simulink model "Polynominal"  (R2019b)
settings: Solver=ode1  StartTime=0.0  StopTime=Inf  FixedStep=0.001  RelTol=1e-3
PostLoadFcn:
  | , if any(exist('dsrtsu_mdlpostloadfcn', 'file') == [2, 3, 6]), try dsrtsu_mdlpostloadfcn('Execute', bdroot); catch fprintf('Error in PostLoadFcn (dsrtsu_mdlpostloadfcn) for model "%s":\n %s\n', bdroot, lasterr); end, end,
Description:
  | Standard RTI1401 template.
  | Supported MATLAB version:  R2018b.
settings Model: Tag=RTI1401  DSRTSU_INTERNAL_RTI_VER=540  DSRTSU_INTERNAL_RTI_TYPE=rti1401  RTICANMMDATA=struct('GeneralSetupData',struct('modelroot','C:\Users\linqi\Desktop\matlab\ACC\CarMaker\src_cm4sl','generalsettings',struct('filesettings',struct('destfolder',struct('Name','RTICANMM_FILES','Check',1),'buildfolder',struct('Name','.','Check',1),'AbsDestfolder',struct('Name','C:\Users\linqi\Desktop\matlab\ACC\CarMaker\src_cm4sl\RTICANMM_FILES'),'AbsBuildfolder',struct('Name','C:\Users\linqi\Desktop\matlab\ACC\CarMaker\src_cm4sl'))),'options',struct('addpaths',1,'rmpaths',1,'addtrcexclusion',logical(1),'cannavigator',struct('checkmonitoring',0),'show_usrtrc',0,'use_usrtrc',0),'advanced',struct('options',ones(1,100)),'MPSetup',{{}},'RTI',struct('Type','RTI1401','Ver','7.12','Date','02-May-2019'),'modelname','','block','untitled'))  DSRTSU_INTERNAL_RTIFPGA=130  Creator=linqi  LastModifiedBy=lenovo
settings DataIOCC: ReturnWorkspaceOutputs=off
settings OptimizationCC: BlockReduction=off  OptimizeBlockIOStorage=off  BufferReuse=off  GlobalBufferReuse=off  ExpressionFolding=off  LocalBlockOutputs=off  OptimizeDataStoreBuffers=off  BusAssignmentInplaceUpdate=off
settings DebuggingCC: ArithmeticOperatorsInVariantConditions=warning
settings HardwareCC: ProdBitPerPointer=32  ProdBitPerSizeT=32  ProdBitPerPtrDiffT=32  ProdLargestAtomicInteger=Integer  ProdEndianess=BigEndian  ProdWordSize=32  ProdHWDeviceType=Custom Processor->Custom  TargetIntDivRoundTo=Zero  TargetEndianess=BigEndian  TargetHWDeviceType=Custom Processor->Custom
settings SFSimCC: SimUseLocalCustomCode=off  MATLABDynamicMemAlloc=off  CustomCodeUndefinedFunction=UseInterfaceOnly
settings RTWCC: Description=dSPACE DS1401 Hardware Platform  SystemTargetFile=rti1401.tlc  MakeCommand=make_rti  TemplateMakefile=rti1401.tmf  RTWUseLocalCustomCode=off
settings CodeAppCC: StateflowObjectComments=on
settings STFCustomTargetCC: ParMdlRefBuildCompliant=on  MatFileLogging=on  SystemTargetFile=rti1401.tlc
settings GRTTargetCC: TargetLangStandard=C89/C90 (ANSI)  CompOptLevelCompliant=off  ConcurrentExecutionCompliant=off  CombineOutputUpdateFcns=off  CPPClassGenCompliant=off  UseToolchainInfoCompliant=off
settings ConfigComp: CovMetricSettings=dswe

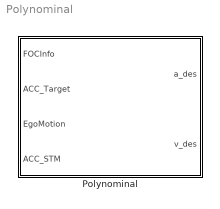
== system Polynominal ==
  Polynominal : Subsystem

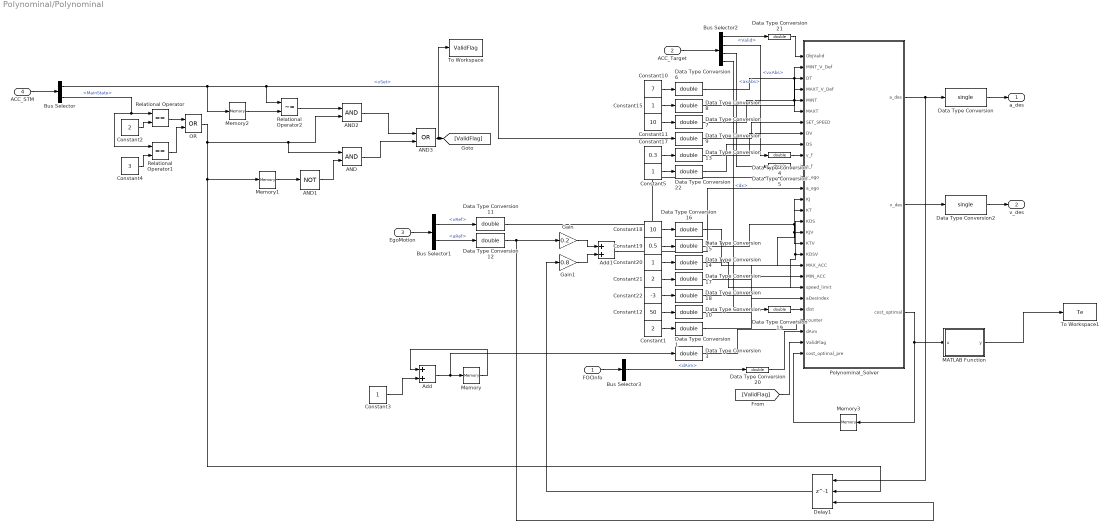
== system Polynominal/Polynominal ==
  FOCInfo : Inport
  ACC_Target : Inport  Port=2
  EgoMotion : Inport  Port=3
  ACC_STM : Inport  Port=4
  AND : Logic  AllPortsSameDT=off  OutDataTypeStr=boolean
  AND1 : Logic  Operator=NOT  AllPortsSameDT=off  OutDataTypeStr=boolean
  AND2 : Logic  AllPortsSameDT=off  OutDataTypeStr=boolean
  AND3 : Logic  Operator=OR  AllPortsSameDT=off  OutDataTypeStr=boolean
  Add : Sum
  Add1 : Sum
  Bus Selector : BusSelector  OutputSignals=vSet,MainState
  Bus Selector1 : BusSelector  OutputSignals=vRef,aRef
  Bus Selector2 : BusSelector  OutputSignals=Valid,vxAbs,axAbs,dx
  Bus Selector3 : BusSelector  OutputSignals=dAim
  Constant1 : Constant  Value=2  OutDataTypeStr=single
  Constant10 : Constant  Value=7  OutDataTypeStr=single
  Constant11 : Constant  Value=10  OutDataTypeStr=single
  Constant12 : Constant  Value=50  OutDataTypeStr=single
  Constant{3,5,15,20} (4 alike) : Constant  OutDataTypeStr=single
  Constant17 : Constant  Value=0.3  OutDataTypeStr=single
  Constant18 : Constant  Value=10  OutDataTypeStr=single
  Constant19 : Constant  Value=0.5  OutDataTypeStr=single
  Constant2 : Constant  Value=2  OutDataTypeStr=single
  Constant21 : Constant  Value=2  OutDataTypeStr=single
  Constant22 : Constant  Value=-3  OutDataTypeStr=single
  Constant4 : Constant  Value=3  OutDataTypeStr=single
  Data Type Conversion : DataTypeConversion  OutDataTypeStr=single
  Data Type Conversion{1,3..22} (21 alike) : DataTypeConversion  OutDataTypeStr=double
  Data Type Conversion2 : DataTypeConversion  OutDataTypeStr=single
  Delay1 : Delay  DelayLength=1  InitialConditionSource=Input port  ExternalReset=Rising
      settings: InputPortMap=u0,r5,p4
  Gain : Gain  Gain=0.2
  Gain1 : Gain  Gain=0.8
  MATLAB Function : MATLAB Function  TreatAsAtomicUnit=on
  Memory : Memory
  Memory1 : Memory
  Memory2 : Memory
  Memory3 : Memory  InitialCondition=zeros(1,12)
  OR : Logic  Operator=OR  AllPortsSameDT=off  OutDataTypeStr=boolean
  Polynominal_Solver : MATLAB Function  TreatAsAtomicUnit=on
  Relational Operator : RelationalOperator  Operator===  OutDataTypeStr=boolean  RndMeth=Simplest
  Relational Operator1 : RelationalOperator  Operator===  OutDataTypeStr=boolean  RndMeth=Simplest
  Relational Operator2 : RelationalOperator  Operator=~=  OutDataTypeStr=boolean  RndMeth=Simplest
  To Workspace : ToWorkspace  VariableName=ValidFlag  SaveFormat=Timeseries  SampleTime=-1
  To Workspace1 : ToWorkspace  VariableName=Te  SaveFormat=Timeseries  SampleTime=-1
  a_des : Outport  VectorParamsAs1DForOutWhenUnconnected=off
  v_des : Outport  Port=2  VectorParamsAs1DForOutWhenUnconnected=off
  wires:
  Bus Selector/1 -> Memory2/1, Relational Operator2/1, Data Type Conversion9/1  "<vSet>"
  Constant12/1 -> Data Type Conversion10/1
  Constant22/1 -> Data Type Conversion18/1
  Constant19/1 -> Data Type Conversion15/1
  Data Type Conversion17/1 -> Polynominal_Solver/20(MAX_ACC)
  Data Type Conversion14/1 -> Polynominal_Solver/16(KDS), Polynominal_Solver/19(KDSV)
  Data Type Conversion10/1 -> Polynominal_Solver/22(speed_limit)
  Data Type Conversion18/1 -> Polynominal_Solver/21(MIN_ACC)
  Constant17/1 -> Data Type Conversion13/1
  Constant20/1 -> Data Type Conversion14/1
  Data Type Conversion7/1 -> Polynominal_Solver/6(MAXT), Polynominal_Solver/4(MAXT_V_Def)
  Data Type Conversion11/1 -> Polynominal_Solver/12(v_ego)
  Constant21/1 -> Data Type Conversion17/1
  Bus Selector1/2 -> Data Type Conversion12/1  "<aRef>"
  Data Type Conversion6/1 -> Polynominal_Solver/5(MINT), Polynominal_Solver/2(MINT_V_Def)
  Data Type Conversion15/1 -> Polynominal_Solver/15(KT), Polynominal_Solver/18(KTV)
  Constant15/1 -> Data Type Conversion8/1
  Constant18/1 -> Data Type Conversion16/1
  Constant11/1 -> Data Type Conversion7/1
  Data Type Conversion9/1 -> Polynominal_Solver/7(SET_SPEED)
  Constant10/1 -> Data Type Conversion6/1
  Data Type Conversion13/1 -> Polynominal_Solver/8(DV)
  Data Type Conversion8/1 -> Polynominal_Solver/3(DT)
  Data Type Conversion16/1 -> Polynominal_Solver/14(KJ), Polynominal_Solver/17(KJV)
  Data Type Conversion12/1 -> Delay1/3, Gain/1
  Polynominal_Solver/1(a_des) -> Delay1/1, Data Type Conversion/1
  ACC_STM/1 -> Bus Selector/1
  EgoMotion/1 -> Bus Selector1/1
  Bus Selector1/1 -> Data Type Conversion11/1  "<vRef>"
  Data Type Conversion/1 -> a_des/1
  Constant1/1 -> Data Type Conversion1/1
  Data Type Conversion1/1 -> Polynominal_Solver/23(aDesIndex)
  Data Type Conversion2/1 -> v_des/1
  Polynominal_Solver/2(v_des) -> Data Type Conversion2/1
  Delay1/1 -> Gain1/1
  Memory/1 -> Add/1
  Constant3/1 -> Add/2
  Add/1 -> Data Type Conversion3/1, Memory/1
  Data Type Conversion3/1 -> Polynominal_Solver/25(counter)
  Bus Selector/2 -> Relational Operator/1, Relational Operator1/1  "<MainState>"
  Constant2/1 -> Relational Operator/2
  Constant4/1 -> Relational Operator1/2
  Relational Operator/1 -> OR/1
  Relational Operator1/1 -> OR/2
  OR/1 -> AND2/2, AND/1, Memory1/1, Delay1/2
  ACC_Target/1 -> Bus Selector2/1
  Bus Selector2/4 -> Data Type Conversion19/1  "<dx>"
  Data Type Conversion4/1 -> Polynominal_Solver/10(v_f)
  Bus Selector2/2 -> Data Type Conversion4/1  "<vxAbs>"
  Data Type Conversion5/1 -> Polynominal_Solver/11(a_f)
  Data Type Conversion19/1 -> Polynominal_Solver/24(dist)
  Data Type Conversion20/1 -> Polynominal_Solver/26(dAim)
  FOCInfo/1 -> Bus Selector3/1
  Bus Selector3/1 -> Data Type Conversion20/1  "<dAim>"
  Gain/1 -> Add1/1
  Gain1/1 -> Add1/2
  Add1/1 -> Polynominal_Solver/13(a_ego)
  Bus Selector2/1 -> Data Type Conversion21/1  "<Valid>"
  Data Type Conversion21/1 -> Polynominal_Solver/1(ObjValid)
  Memory1/1 -> AND1/1
  AND1/1 -> AND/2
  Memory2/1 -> Relational Operator2/2
  Relational Operator2/1 -> AND2/1
  AND2/1 -> AND3/1
  AND/1 -> AND3/2
  AND3/1 -> To Workspace/1, [ValidFlag]
  [ValidFlag] -> Polynominal_Solver/27(ValidFlag)
  Memory3/1 -> Polynominal_Solver/28(cost_optimal_pre)
  Polynominal_Solver/3(cost_optimal) -> MATLAB Function/1(u), Memory3/1
  MATLAB Function/1(y) -> To Workspace1/1
  Constant5/1 -> Data Type Conversion22/1
  Data Type Conversion22/1 -> Polynominal_Solver/9(DS)
  Bus Selector2/3 -> Data Type Conversion5/1  "<axAbs>"

== matlab function Polynominal/Polynominal_Solver ==
  data: ObjValid input; MINT_V_Def input; a_des output; DT input; MAXT_V_Def input; MINT input; MAXT input; SET_SPEED input; DV input; DS input; v_f input; a_f input; v_ego input; a_ego input; KJ input; KT input; KDS input; KJV input; KTV input; KDSV input; MAX_ACC input; MIN_ACC input; speed_limit input; aDesIndex input; v_des output; dist input; counter input; dAim input; ValidFlag input; cost_optimal output; cost_optimal_pre input
function [a_des,v_des,cost_optimal] = ACC_PLANNING(ObjValid, MINT_V_Def,DT,MAXT_V_Def, MINT,MAXT,SET_SPEED,DV,DS,v_f,a_f,v_ego,a_ego,KJ,KT,KDS,KJV, KTV, KDSV,MAX_ACC, MIN_ACC,speed_limit,aDesIndex,...
    dist,counter, dAim,ValidFlag, cost_optimal_pre)
        breakTrig = 0;
        s_of_t = zeros(200,1);
        v_of_t = zeros(200,1);
        a_of_t = zeros(200,1);
        t_data = zeros(200,1);
        a_des = 0;
        v_des = 0;
        cost_optimal = zeros(1,12);
if counter <= 250
    breakTrig = 0;
else
    breakTrig = 1;
end        
    if ObjValid == 0
% No valid Object, Set Speed Control uses traditional PID controller.
% Following planning based controller is no longer used.
%         [MINT_V,MAXT_V] = calcTimeSampleOfV(v_ego,MINT_V_Def,MAXT_V_Def,ValidFlag,cost_optimal_pre);
%         [cost_graph] = cal_velocity_control(MINT_V,DT,MAXT_V, SET_SPEED,DV,v_ego, a_ego, KJV, KTV, KDSV); 
%         [cost_optimal] = check_quantic_status(cost_graph,speed_limit, MAX_ACC, MIN_ACC,MAXT_V); 
%         [s_of_t, v_of_t,a_of_t, t_data] = combination_quantic(cost_optimal); 
%         a_des = min(max(a_of_t(aDesIndex),-1.5),1.5);
%         v_des = min(max(v_of_t(2),0),speed_limit);
        a_des = 16;
        v_des = SET_SPEED;
        
        
    else
        D0 = 0; % ONLY for test convenience
        TTC = 0;
        
        [cost_graph] = cal_distance_control(MINT,DT,MAXT,v_f,a_f,dist,D0,TTC,DS,v_ego,a_ego,KJ,KT,KDS,dAim);
        cost_optimal = check_status(cost_graph,speed_limit, MAX_ACC, MIN_ACC,MAXT);
        [s_of_t, v_of_t,a_of_t, t_data] = combination_quintic(cost_optimal);
        a_des = min(max(a_of_t(aDesIndex),-4),1.5);
        v_des = min(max(v_of_t(2),0),speed_limit);
    end
    
    
end


    


function [cost_graph] = cal_distance_control(MINT,DT,MAXT,v_f,a_f,dist,D0,TTC,DS,v_pre,a_pre,KJ,KT,KDS,dAim)
    
    cost_graph = ones(400,12)* 500; 
    index = 1;
    tStopMethod = 2;
    for Ti = MINT : DT : MAXT
        tStop = cal_tStop(v_f,a_f,Ti,tStopMethod);
        [dist_t] = cal_dist_t(dist,v_f,a_f,Ti,tStop,tStopMethod);
        v_f_t = cal_v_f_t(v_f, a_f, Ti,tStop,tStopMethod);
        %[s_des] = cal_s_des(D0, TTC, v_f_t);
        s_des = dAim;
        [s_target] = cal_s_target(s_des,dist_t);
        [s_target_d] = cal_s_target_d(v_f_t, TTC, a_f);
        [s_target_dd] = cal_s_target_dd(v_f,a_f, Ti,tStop, tStopMethod);
        delta_s = 0.25 * abs(s_target);
        
        for Si = (s_target - delta_s) : DS : (s_target + delta_s) 
            s0 = 0;
            v0 = v_pre;
            a0 = a_pre;
            se = Si;
            ve = s_target_d;
            ae = s_target_dd;
            [a0, a1, a2, a3, a4,a5] = quintic_polynomial(s0, ...
                v0, a0, se, ve, ae,Ti);
            %get the quintic polu parameters;
            [jerk,count] = cal_jerk(a3,a4,a5,Ti);
            cost_J = mean(abs(jerk(1:count)));
            cost_T = Ti;
            cost_DS = sqrt((s_target - Si)^2);
            cost_total = KJ * cost_J + KT * cost_T + KDS * cost_DS;
            cost_graph(index,:) = [cost_total,Ti,Si,cost_J,cost_T,cost_DS,...
                a0, a1, a2, a3, a4, a5];
            
            index = index + 1;
        end
    end
    cost_graph = sortrows(cost_graph);
end

function [cost_graph] = cal_velocity_control(MINT_V,DT,MAXT_V, SET_SPEED,DV,v_pre, a_pre, KJV, KTV, KDSV)
    cost_graph = ones(400,11)* 500;    
    index = 1;
    delta_v = 0.1 * SET_SPEED;

    for Ti = MINT_V : DT : MAXT_V
        for Ve = SET_SPEED - 0.3 : DV : SET_SPEED + 0.3
            s0 = 0;
            v0 = v_pre;
            a0 = a_pre;
            ve = Ve;
            ae = 0;
            [a0, a1, a2, a3, a4] = quantic_polynomial(s0, ...
                v0, a0, ve, ae,Ti);
            [jerk,count] = cal_quantic_jerk(a3,a4,Ti);
            cost_J = mean(abs(jerk(1:count)));
            cost_T = Ti;
            cost_DV = sqrt((SET_SPEED - Ve)^2);
            cost_total = KJV * cost_J + KTV * cost_T + KDSV * cost_DV;
            cost_graph(index,:) = [cost_total,Ti,Ve,cost_J,cost_T,cost_DV,...
                a0, a1, a2, a3, a4];

            index = index + 1;
        end
    end
    cost_graph = sortrows(cost_graph);
end

function [cost_optimal] = check_status(cost_graph,speed_limit, MAX_ACC, MIN_ACC,MAXT)
    i = 1;
    COND = 1;
    cost_optimal = zeros(1,12);
    LEN_T = 0;
    
    if isempty(cost_graph)
        cost_optimal=  zeros(1,12);
        fprintf("error in cost graph.");
        return;
    end
    
    valid_range = find(cost_graph(:,2) == 500);
    valid_size = valid_range(1);
    
    while COND == 1
        

        
        poly_para = cost_graph(i,7:12);
        a0 = poly_para(1); a1 = poly_para(2); a2 = poly_para(3); 
        a3 = poly_para(4); a4 = poly_para(5); a5 = poly_para(6);
        
        Te = cost_graph(i,2);
        LEN_T = double(Te * 5 + 1);
        vt = zeros(200,1);
        at = zeros(200,1);
        
        
        for j = 1: LEN_T
            t = (j-1) * 0.2;
            vt(j) = calc_first_derivative(a1,a2,a3,a4,a5,t);
            at(j) =  calc_second_derivative(a2,a3,a4,a5,t);
        end
        
        if cost_graph(i,1) == 500
            COND = 2;
        end
        
        
        
        
        if (max(abs(vt)) <= speed_limit && max(at) <= MAX_ACC && min(at) >= MIN_ACC)
            cost_optimal = cost_graph(i,:);
            COND = 2;
        end
        
        i = i + 1;
        
        if i == valid_size
            COND = 2;
            POS = find(cost_graph(:,2) == MAXT);
            POS_first = POS(1); % find the first combination with longest T; 
            cost_optimal = cost_graph(POS_first,:);
        end
    end
end

function [cost_optimal] = check_quantic_status(cost_graph,speed_limit, MAX_ACC, MIN_ACC,MAXT_V)
    i = 1;
    COND = 1;
    cost_optimal = zeros(1,12);
    LEN_T = 0;
    
    if isempty(cost_graph)
        cost_optimal=  zeros(1,12);
        fprintf("error in cost graph.");
        return;
    end
    
    valid_range = find(cost_graph(:,2) == 500);
    valid_size = valid_range(1);

    while COND == 1

        
        poly_para = cost_graph(i,7:11);
        a0 = poly_para(1); a1 = poly_para(2); a2 = poly_para(3); 
        a3 = poly_para(4); a4 = poly_para(5); 
        
        Te = cost_graph(i,2);
        
        LEN_T = double(Te * 5 + 1);
        vt = zeros(200,1);
        at = zeros(200,1);
        
        for j = 1: LEN_T
            t = (j-1) * 0.2;
            vt(j) = calc_quantic_first_derivative(a1,a2,a3,a4,t);
            at(j) = calc_quantic_second_derivative(a2,a3,a4,t);
        end
        
        
        if cost_graph(i,1) == 500
            COND = 2;
        end
        
        if (max(abs(vt)) <= speed_limit && max(at) <= MAX_ACC && min(at) >= MIN_ACC)
            cost_optimal(1:11) = cost_graph(i,:);
            COND = 2;
        end
        
        i = i + 1;
        
        if i == valid_size
            COND = 2;
            POS = find(cost_graph(:,2)==MAXT_V);
            POS_first = POS(1); % find the first combination with longest T; 
            cost_optimal(1:11)  = cost_graph(POS_first,:);
        end
    end
end

function [a0, a1, a2, a3, a4] = quantic_polynomial(xs, ...
    vxs, axs, vxe, axe,T)
    
    A  =[1,0,0,0,0;0,1,0,0,0;0,0,2,0,0;...
        0,1,2*T,3*T^2,4*T^3;0,0,2,6*T,12*T^2];
    
    if det(A) == 0
        a0 = [];
        a1 = [];
        a2 = [];

        a3 = [];
        a4 = [];


        fprintf('cannot calculate quintic polynomial paras.');
        return;
    end
    
    
    b = [xs,vxs,axs,vxe,axe]';
    x = pinv(A) * b;
    
    a0 = x(1);
    a1 = x(2);
    a2 = x(3);
    a3 = x(4);
    a4 = x(5);
end

function [a0, a1, a2, a3, a4,a5] = quintic_polynomial(xs, ...
    vxs, axs, xe, vxe, axe,T)
% A = [0,0,0,0,0,1; T^5,T^4,T^3,T^2,T,1;...
%     0,0,0,0,1,0 ; 5*T^4  4*T^3 3*T^2 2*T 1 0 ; ...
%     0 0 0 2 0 0; 20*T^3 12*T^2 6*T 2 0 0];
% b = [xs, xe, vxs, vxe, axs, 0]';
% x = A\b;
% a5 = x(1);
% a4 = x(2);
% a3 = x(3);
% a2 = x(4);
% a1 = x(5);
% a0 = x(6);
A = [T^3 T^4 T^5; 3*T^2 4*T^3 5*T^4; 6*T 12*T^2 20*T^3];
b = [(xe - xs  - vxs*T - 0.5*axs*T^2); (vxe- vxs - axs*T ); (axe - axs)];

if det(A) == 0
    a0 = [];
    a1 = [];
    a2 = [];

    a3 = [];
    a4 = [];
    a5 = [];  
    
    fprintf('cannot calculate quintic polynomial paras.');
    return;
end


    
    
x = pinv(A) * b;
a0 = xs;
a1 = vxs;
a2 = axs/2;

a3 = x(1);
a4 = x(2);
a5 = x(3);
end

function [jerk,count] = cal_jerk(a3,a4,a5,Ti)
    seg = 15 / 0.1 + 1;
    count = Ti / 0.1 + 1;
    index = 1;
    jerk = zeros(1,seg);
    
    for k = 1:count
        i  = k * 0.1;
        jerk(index) =  6* a3  + 24 * a4 * i + 60* a5 *i^2;
        index = index + 1;
    end
end

function [jerk,count] = cal_quantic_jerk(a3,a4,Ti)
    seg = 15 / 0.1 + 1;
    count = floor(Ti / 0.1 + 1);
    index = 1;
    jerk = zeros(1,seg);
    
    for k = 1:count
        i  = k * 0.1;
        jerk(index) =  6* a3 + 24 * a4 * i;
        index = index + 1;
    end
end

function [s_of_t, v_of_t,a_of_t, t_data] = combination_quintic(cost_optimal)
    if isempty(cost_optimal)
        s_of_t = zeros(200,1);
        v_of_t = zeros(200,1);
        t_data = zeros(200,1);
        fprintf("error in optimal cost graph.");
        return;
    end

   
    Te = cost_optimal(2);
    poly_para = cost_optimal(7:12);
    a0 = poly_para(1); a1 = poly_para(2); a2 = poly_para(3); 
    a3 = poly_para(4); a4 = poly_para(5); a5 = poly_para(6);
   s_of_t = zeros(200,1);
    v_of_t = zeros(200,1);
    a_of_t = zeros(200,1);
    t_data = zeros(200,1);
    
    index = 1;
    seg = Te / 0.1 - 1;
    
    for i = 0 : seg
        t = i * 0.1;
        s_of_t(index) = calc_point(a0,a1,a2,a3,a4,a5,t);
        v_of_t(index) = calc_first_derivative(a1,a2,a3,a4,a5,t);
        a_of_t(index) =  calc_second_derivative(a2,a3,a4,a5,t);
        t_data(index) = t;
        index = index + 1;
    end
end

function [s_of_t, v_of_t,a_of_t,t_data] = combination_quantic(cost_optimal)
    if isempty(cost_optimal)

        fprintf("error in optimal cost graph.");
        return;
    end

    Te = cost_optimal(2);
    poly_para = cost_optimal(7:11);
    a0 = poly_para(1); a1 = poly_para(2); a2 = poly_para(3); 
    a3 = poly_para(4); a4 = poly_para(5); 
    s_of_t = zeros(200,1);
    v_of_t = zeros(200,1);
    a_of_t = zeros(200,1);
    t_data = zeros(200,1);
    
    index = 1;
    seg = Te / 0.1 - 1;
    
    for i = 0 : seg
        t = i * 0.1;
        s_of_t(index) = cal_quantic_point(a0,a1,a2,a3,a4,t);
        v_of_t(index) = calc_quantic_first_derivative(a1,a2,a3,a4,t);
        a_of_t(index) = calc_quantic_second_derivative(a2,a3,a4,t);
        t_data(index) = t;
        index = index + 1;
    end
end


function [xt] = calc_point(a0,a1,a2,a3,a4,a5,T)
    xt = a0 + a1 * T + a2 * T^2 + a3 * T^3 + a4 * T^4 + a5 * T^5;
end

function [xt] = cal_quantic_point(a0,a1,a2,a3,a4,T)
    xt = a0 + a1 * T + a2 * T^2 + a3 * T^3 + a4 * T^4;
end

function [xt] =calc_first_derivative(a1,a2,a3,a4,a5,t)
xt = a1 + 2 * a2 * t + 3 * a3 * t^2 + 4 * a4 * t^3 + 5 * a5 * t^4;
end

function [xt]  = calc_second_derivative(a2,a3,a4,a5,t)
xt = 2* a2 + 6* a3 * t + 12 * a4 * t^2 + 20* a5 *t^3;
end

function [xt] =calc_quantic_first_derivative(a1,a2,a3,a4,t)
xt = a1 + 2 * a2 * t + 3 * a3 * t^2 + 4 * a4 * t^3;
end

function [xt]  = calc_quantic_second_derivative(a2,a3,a4,t)
xt = 2* a2 + 6* a3 * t + 12 * a4 * t^2;
end

function a_f_t = cal_a_f_t(v_f,a_f, Ti,tStop)
    if tStop == 0
        a_f_t = 0;
    else
        a_f_d = -a_f/min(Ti,tStop);    
        a_f_t = a_f + a_f_d * min(Ti,tStop);
    end
end
function v_f_t = cal_v_f_t(v_f, a_f, Ti,tStop,tStopMethod)
    %calculate v_f of time.
if tStopMethod == 1
    if tStop == 0
        a_f_d = 0;
    else
        a_f_d = -a_f/min(Ti,tStop);
    end
    v_f_t = v_f + a_f * min(Ti,tStop)+0.5*a_f_d*min(Ti,tStop)^2;
elseif tStopMethod == 2
    t = min(Ti,tStop);
    T = Ti/2.3;
    v_f_t = -a_f*T*exp(-t/T) + v_f + a_f*T;
else
    
end
    
end

function [dist_t] = cal_dist_t(dist,v_f,a_f,Ti,tStop,tStopMethod)
    %calculate distance of time.
if tStopMethod == 1
    if tStop == 0
        a_f_d = 0;
    else
    a_f_d = -a_f/min(Ti,tStop);
    end
    
    if tStop >= Ti
        dist_t = dist + v_f * Ti + 1/2 * a_f * Ti^2 + 1/6 * a_f_d * Ti^3;
%           dist_t = dist + (v_f + a_f*tElapes)*Ti + a_f*tElapes^2*exp(-Ti/tElapes) - a_f*tElapes^2;
    else
        dist_t = dist + v_f * tStop + 1/2 * a_f * tStop^2 + 1/6 * a_f_d * tStop^3;
    end
elseif tStopMethod == 2  
    T = Ti/2.3;
    t = min(tStop,Ti);
    dist_t = dist + (v_f+a_f*T)*t + a_f*T^2*exp(-t/T) - a_f*T^2;
else
    
end
    
end


function [s_des] = cal_s_des(D0, TTC, v_f_t)
    %calculate desired s.
%     s_des = D0 + TTC * v_f_t;
     s_des = 20; % here we made a simplification
end


function [s_target] = cal_s_target(s_des,dist_t)
    %calculate s target.
    s_target = dist_t - s_des;
end

function [s_target_d] = cal_s_target_d(v_f_t, TTC, a_f)
    %calculate v_f of time.
%     s_target_d = v_f_t - TTC * a_f;
    s_target_d = v_f_t; % here we made a simplification
end


function [s_target_dd] = cal_s_target_dd(v_f,a_f, Ti,tStop, tStopMethod)
if tStopMethod == 1
    a_f_d = cal_a_f_t(v_f,a_f, Ti,tStop);
    s_target_dd =    a_f +   a_f_d *  min(Ti,tStop);   
elseif tStopMethod == 2
    if tStop < Ti
        s_target_dd = 0;
    else
        T = Ti/2.3;
        s_target_dd = a_f * exp(-Ti/T);
    end
else
    
end
end

function [y] = LinearInterpolation(X,Y,x)
    % input: X, Y, x
    % output: y
    % breif: in a matrix [X,Y] , input any x in range of X, to search
    % respective y in range of Y.
    y = 0;    
    if isempty(X)
            y = 0;
    end
    
    low = 1;
    high = length(X);
    
    if x <= X(low) 
        y = Y(low);
        return;
    end
    
    if x >= X(high)
        y = Y(high);
        return;
    end

    Flag = 0;
    
    while Flag == 0
        mid = round(0.5 * (low + high));
        if x == X(mid)
            y = Y(mid);
            Flag = 1;
            break;
            
        elseif x < X(mid)
            high =  mid;
        else
            low = mid;
        end
        
        if (high - low) == 1
            Flag = 1;
        end
       y = Y(low)  + (x - X(low))/(X(high) - X(low)) * (Y(high) - Y(low));
 
    end
    
end

function [MINT_V,MAXT_V] = calcTimeSampleOfV(vRef,MINT_V_Def,MAXT_V_Def,ValidFlag,cost_optimal_pre)
    if ValidFlag == 1
        MINT_V = MINT_V_Def;
        MAXT_V = MAXT_V_Def;
    else
        Te = cost_optimal_pre(2);
%         poly_para = cost_optimal_pre(7:11);
%         a0 = poly_para(1); a1 = poly_para(2); a2 = poly_para(3); 
%         a3 = poly_para(4); a4 = poly_para(5); 
%         v_of_t = zeros(200,1);
%         t_data = zeros(200,1);
%         index = 1;
%         seg = Te / 0.1 - 1;
%         for i = 0 : seg
%             t = i * 0.1;
%             v_of_t(index) = calc_quantic_first_derivative(a1,a2,a3,a4,t);
%             t_data(index) = t;
%             index = index + 1;
%         end
        
        tReal = Te-0.02;
        MINT_V = max(3,tReal);
        MAXT_V = MINT_V;
    end
end

function [tStop] = cal_tStop(v_f,a_f,Ti,tStopMethod)
    % constant Jerk Prediction Model(cJPM):tStopMethod == 1
    % Exponetial Prediction Model(EPM):tStopMethod == 2
    if (tStopMethod == 1)
        if (a_f>=0)
            tStop = 255;
        else if v_f <= 0
              tStop = 0;  
        else
            a_f_d = (0-a_f)/Ti;
            v_f_Ti = v_f + a_f * Ti + 1/2 * a_f_d * Ti^2;
            if v_f_Ti > 0
                tStop = 255;
            else
                a = 1/2 * a_f_d;
                b = a_f;
                c = v_f;
                tRoot1 = (-b + sqrt(b^2-4*a*c))/(2*a);
                tRoot2 = (-b - sqrt(b^2-4*a*c))/(2*a);
                tRoot = min(tRoot1,tRoot2);
                if tRoot <= Ti
                    tStop = tRoot;
                else
                    tStop = 255;
                end
            end
            end
        end
    elseif(tStopMethod == 2)
        T = Ti/2.3;
        if (a_f>=0)
            tStop = 255;
        else if v_f <= 0
              tStop = 0;  
        else

            v_f_Ti = -a_f*T*exp(-Ti/T)+v_f+a_f*T;
            if v_f_Ti > 0
                tStop = 255;
            else
                tStop = -T*log((v_f+a_f*T)/(a_f*T));
            end
            end
        end
    else
        
    end
    
end

== matlab function Polynominal/MATLAB Function ==
  data: u input; y output
function y = fcn(u)

y = u(2);
